simulink model "base"  (R2025b)
settings: Solver=VariableStepAuto  StartTime=0.0  StopTime=10.0  RelTol=1e-3
settings Model: Creator=Utente  LastModifiedBy=Utente

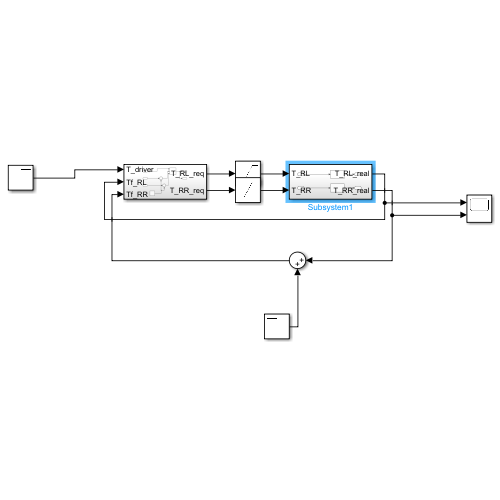
[thumbnail: Simulink's stored preview of the top-level diagram]
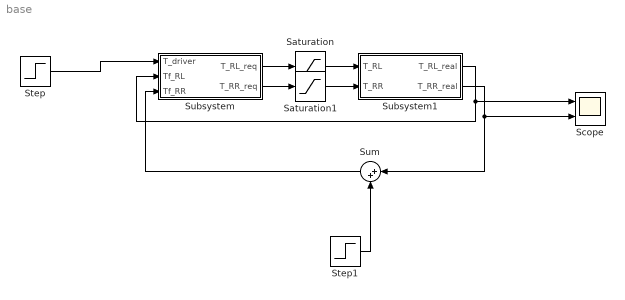
== system base ==
  Saturation : Saturate  UpperLimit=21  LowerLimit=-21
  Saturation1 : Saturate  UpperLimit=21  LowerLimit=-21
  Scope : Scope  NumInputPorts=2
      settings: ActiveDisplayYMinimum=-1.3781420674651468  ActiveDisplayYMaximum=25.905071323596172
  Step : Step  Time=2  After=21  SampleTime=0
  Step1 : Step  Time=6  After=-10  SampleTime=0
  Subsystem : Subsystem
  Subsystem1 : Subsystem
  Sum : Sum  Inputs=|++
  wires:
  Step/1 -> Subsystem/1(T_driver)
  Step1/1 -> Sum/2
  Subsystem1/2(T_RR_real) -> Sum/1, Scope/2
  Sum/1 -> Subsystem/3(Tf_RR)
  Subsystem1/1(T_RL_real) -> Subsystem/2(Tf_RL), Scope/1
  Subsystem/1(T_RL_req) -> Saturation/1
  Subsystem/2(T_RR_req) -> Saturation1/1
  Saturation/1 -> Subsystem1/1(T_RL)
  Saturation1/1 -> Subsystem1/2(T_RR)

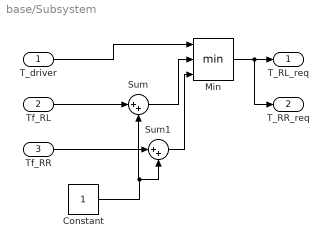
== system base/Subsystem ==
  T_driver : Inport
  Tf_RL : Inport  Port=2
  Tf_RR : Inport  Port=3
  Constant : Constant
  Min : MinMax  Inputs=3
  Sum : Sum  Inputs=|++
  Sum1 : Sum  Inputs=|++
  T_RL_req : Outport
  T_RR_req : Outport  Port=2
  wires:
  Tf_RR/1 -> Sum1/1
  Constant/1 -> Sum/2, Sum1/2
  Tf_RL/1 -> Sum/1
  T_driver/1 -> Min/1
  Sum/1 -> Min/2
  Sum1/1 -> Min/3
  Min/1 -> T_RR_req/1, T_RL_req/1

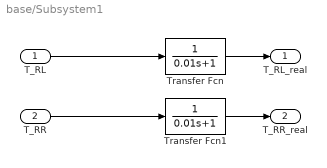
== system base/Subsystem1 ==
  T_RL : Inport
  T_RR : Inport  Port=2
  Transfer Fcn : TransferFcn  Denominator=[0.01 1]
  Transfer Fcn1 : TransferFcn  Denominator=[0.01 1]
  T_RL_real : Outport
  T_RR_real : Outport  Port=2
  wires:
  T_RL/1 -> Transfer Fcn/1
  Transfer Fcn/1 -> T_RL_real/1
  Transfer Fcn1/1 -> T_RR_real/1
  T_RR/1 -> Transfer Fcn1/1
